simulink model "SPM_Model"  (R2023a)
settings: Solver=ode3  StartTime=0  StopTime=fin  FixedStep=st  MaxStep=0.5  RelTol=1e-3  EnableMultiTasking=on
values from neighbouring files (symbols this model uses):
  Asys_n = alpha1_n * a_setup    [SPM_Script.m]
  Asys_p = alpha1_p * a_setup    [SPM_Script.m]
  Bsys_n = alpha2_n * [zeros(num-1,1); -sr / (sr - 1)]    [SPM_Script.m]
  Bsys_p = alpha2_p * [zeros(num-1,1); -sr / (sr - 1)]    [SPM_Script.m]
  cs_init_n = x_init * cs_max_n    [SPM_Script.m]    (also in TPM_Script.m = (SOC_p20 * (x100_percent_n - x0_percent_n) + x0_percent_n) *)
  cs_init_p = y_init * cs_max_p    [SPM_Script.m]    (also in TPM_Script.m = (SOC_p20 * (y100_percent_p - y0_percent_p) + y0_percent_p) *)
  Csys_n = [zeros(1, num-1), 1]    [SPM_Script.m]
  Csys_p = [zeros(1, num-1), 1]    [SPM_Script.m]
  Dsys_n = -alpha2_n / alpha1_n    [SPM_Script.m]
  Dsys_p = -alpha2_p / alpha1_p    [SPM_Script.m]
  PA = 5    [SPM_Script.m]    (also in TPM_Script.m)
  par = zeros(11, 1)    [TPM_Script.m]
settings Model: Creator=Cra  LastModifiedBy=srose
settings SolverCC: AlgebraicLoopSolver=TrustRegion
settings DataIOCC: SaveFormat=Array  SignalLoggingSaveFormat=ModelDataLogs  SaveOutput=off  SignalLogging=off  ReturnWorkspaceOutputs=off
settings OptimizationCC: ExpressionDepthLimit=2147483647  InitFltsAndDblsToZero=on  LifeSpan=inf
settings DebuggingCC: SaveWithParameterizedLinksMsg=none  UnderspecifiedInitializationDetection=Classic  MergeDetectMultiDrivingBlocksExec=none  SolverPrmCheckMsg=warning  FcnCallInpInsideContextMsg=warning  UnconnectedInputMsg=warning  UnconnectedOutputMsg=warning  UnconnectedLineMsg=warning  StateNameClashWarn=warning  SFUnexpectedBacktrackingDiag=warning  SFNoUnconditionalDefaultTransitionDiag=warning  SFExecutionAtInitializationDiag=none  ArithmeticOperatorsInVariantConditions=warning
settings HardwareCC: ProdBitPerPointer=32  ProdBitPerSizeT=32  ProdBitPerPtrDiffT=32  ProdLargestAtomicFloat=None  ProdIntDivRoundTo=Undefined  ProdEndianess=Unspecified  ProdWordSize=32  ProdHWDeviceType=32-bit Generic
settings ModelReferenceCC: EnableRefExpFcnMdlSchedulingChecks=on  PropagateSignalLabelsOutOfModel=off
settings SFSimCC: SimUseLocalCustomCode=off  CustomCodeUndefinedFunction=UseInterfaceOnly
settings RTWCC: RTWUseLocalCustomCode=off  DLArmComputeVersion=19.05
settings CodeAppCC: StateflowObjectComments=on
settings GRTTargetCC: TargetFcnLib=ansi_tfl_tmw.mat  TargetLangStandard=C89/C90 (ANSI)  CombineOutputUpdateFcns=off  GRTInterface=on
settings ConfigComp: CovMetricSettings=dw  CovSaveCumulativeToWorkspaceVar=on  CovSaveSingleToWorkspaceVar=on  CovExternalEMLEnable=off

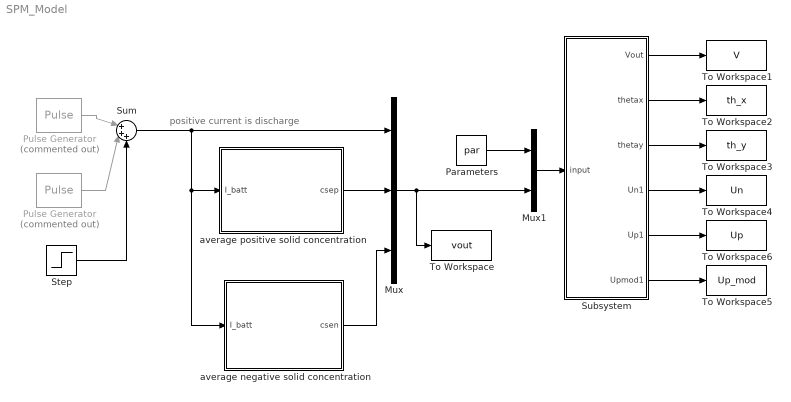
== system SPM_Model ==
  note: positive current is discharge
  Mux : Mux  Inputs=3
  Mux1 : Mux  Inputs=2
  Parameters : Constant  Value=par  VectorParams1D=off
  Pulse Generator : DiscretePulseGenerator  Commented=on  PulseType=Time based  Amplitude=-2*PA  Period=100  PulseWidth=25  PhaseDelay=140
  "Pulse Generator " : DiscretePulseGenerator  Commented=on  PulseType=Time based  Amplitude=PA  Period=100  PulseWidth=25  PhaseDelay=40
  Step : Step  Time=0  After=5  SampleTime=0
  Subsystem : Subsystem
  Sum : Sum  Inputs=|+++
  To Workspace : ToWorkspace  VariableName=vout  SampleTime=-1
  To Workspace1 : ToWorkspace  VariableName=V  SampleTime=-1
  To Workspace2 : ToWorkspace  VariableName=th_x  SampleTime=-1
  To Workspace3 : ToWorkspace  VariableName=th_y  SampleTime=-1
  To Workspace4 : ToWorkspace  VariableName=Un  SampleTime=-1
  To Workspace5 : ToWorkspace  VariableName=Up_mod  SampleTime=-1
  To Workspace6 : ToWorkspace  VariableName=Up  SampleTime=-1
  "average negative solid concentration  " : Subsystem
  average positive solid concentration : Subsystem
  wires:
  average positive solid concentration/1(csep) -> Mux/2
  Mux/1 -> Mux1/2, To Workspace/1
  "average negative solid concentration  "/1(csen) -> Mux/3
  Sum/1 -> average positive solid concentration/1(I_batt), "average negative solid concentration  "/1(I_batt), Mux/1
  "Pulse Generator "/1 -> Sum/1
  Pulse Generator/1 -> Sum/2
  Step/1 -> Sum/3
  Parameters/1 -> Mux1/1
  Mux1/1 -> Subsystem/1(input)
  Subsystem/1(Vout) -> To Workspace1/1
  Subsystem/2(thetax) -> To Workspace2/1
  Subsystem/3(thetay) -> To Workspace3/1
  Subsystem/4(Un1) -> To Workspace4/1
  Subsystem/5(Up1) -> To Workspace6/1
  Subsystem/6(Upmod1) -> To Workspace5/1

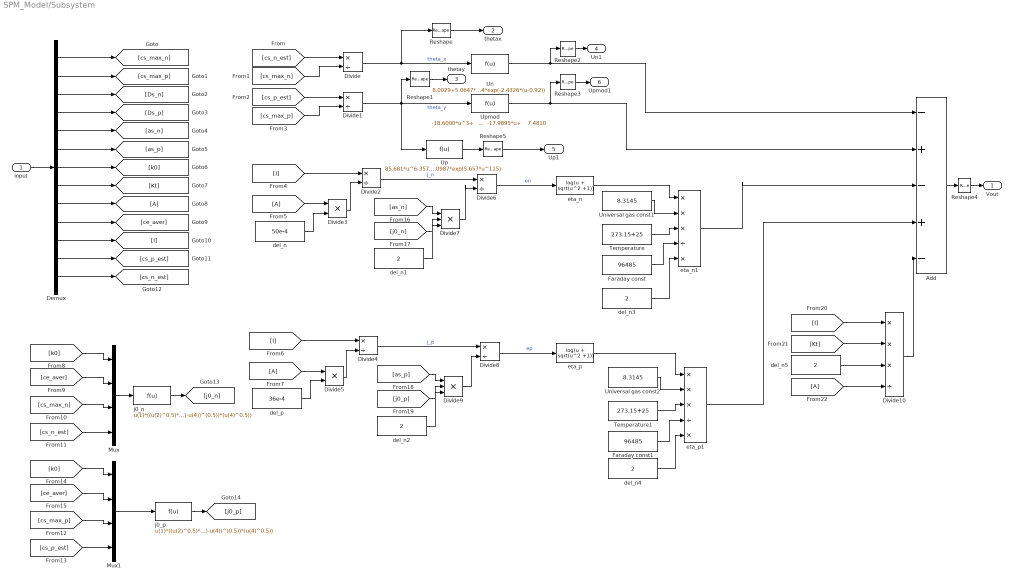
== system SPM_Model/Subsystem ==
  input : Inport
  Add : Sum  Inputs=-+-+-  OutDataTypeStr=double
  Demux : Demux  Outputs=13
  Divide{,1..2,4,6,8} (6 alike) : Product  Inputs=*/
  Divide10 : Product  Inputs=***/
  Divide3 : Product  Inputs=**
  Divide5 : Product  Inputs=**
  Divide7 : Product  Inputs=***
  Divide9 : Product  Inputs=***
  Faraday const : Constant  Value=96485
  Faraday const1 : Constant  Value=96485
  From22 : From
  From5 : From
  From7 : From
  Goto8 : Goto
  Mux : Mux
  Mux1 : Mux
  Reshape{,1..5} (6 alike) : Reshape
  Temperature : Constant  Value=273.15+25
  Temperature1 : Constant  Value=273.15+25
  Un : Fcn  Expr=8.0029+5.0647*u-12.578*u^0.5-8.6322e-4*u^(-1)+2.1765e-5*u^(3/2)-0.46016*exp(15.0*(0.06-u))-0.55364*exp(-2.4326*(u-0.92))
  Universal gas const1 : Constant  Value=8.3145  VectorParams1D=off
  Universal gas const2 : Constant  Value=8.3145
  Up : Fcn  Expr=85.681*u^6-357.70*u^5+613.89*u^4-555.65*u^3+281.06*u^2-76.648*u+13.1983 -0.30987*exp(5.657*u^115)
  Upmod : Fcn  Expr="-18.6000*u^3+   31.1854*u^2  -17.9895*u+    7.4810"
  del_n : Constant  Value=50e-4
  del_n{1..5} (5 alike) : Constant  Value=2
  del_p : Constant  Value=36e-4
  eta_n : Fcn  Expr=log(u + sqrt(u^2 +1))
  eta_n1 : Product  Inputs=***/*
  eta_p : Fcn  Expr=log(u + sqrt(u^2 +1))
  eta_p1 : Product  Inputs=***/*
  j0_n : Fcn  Expr=u(1)*((u(2)^0.5)*((u(3)-u(4))^(0.5))*(u(4)^0.5))
  j0_p : Fcn  Expr=u(1)*((u(2)^0.5)*((u(3)-u(4))^(0.5))*(u(4)^0.5))
  Vout : Outport
  thetax : Outport  Port=2
  thetay : Outport  Port=3
  Un1 : Outport  Port=4
  Up1 : Outport  Port=5
  Upmod1 : Outport  Port=6
  wires:
  input/1 -> Demux/1
  Demux/1 -> [cs_max_n]
  Demux/2 -> [cs_max_p]
  Demux/3 -> [Ds_n]
  Demux/4 -> [Ds_p]
  Demux/5 -> [as_n]
  Demux/6 -> [as_p]
  Demux/7 -> [k0]
  Demux/8 -> [Kt]
  Demux/9 -> Goto8/1
  Demux/10 -> [ce_aver]
  Demux/11 -> [I]
  Demux/12 -> [cs_p_est]
  Demux/13 -> [cs_n_est]
  [cs_n_est] -> Divide/1
  [cs_max_n] -> Divide/2
  Divide/1 -> Un/1, Reshape/1  "theta_x"
  [cs_p_est] -> Divide1/1
  [cs_max_p] -> Divide1/2
  Divide1/1 -> Upmod/1, Up/1, Reshape1/1  "theta_y"
  [I] -> Divide2/1
  From5/1 -> Divide3/1
  del_n/1 -> Divide3/2
  Divide3/1 -> Divide2/2
  Divide2/1 -> Divide6/1  "j_n"
  [I] -> Divide4/1
  From7/1 -> Divide5/1
  del_p/1 -> Divide5/2
  Divide5/1 -> Divide4/2
  Divide4/1 -> Divide8/1  "j_p"
  [k0] -> Mux/1
  [ce_aver] -> Mux/2
  [cs_max_n] -> Mux/3
  [cs_n_est] -> Mux/4
  Mux/1 -> j0_n/1
  [k0] -> Mux1/1
  [ce_aver] -> Mux1/2
  [cs_max_p] -> Mux1/3
  [cs_p_est] -> Mux1/4
  Mux1/1 -> j0_p/1
  [as_n] -> Divide7/1
  [j0_n] -> Divide7/2
  Divide7/1 -> Divide6/2
  j0_n/1 -> [j0_n]
  j0_p/1 -> [j0_p]
  del_n1/1 -> Divide7/3
  [as_p] -> Divide9/1
  [j0_p] -> Divide9/2
  Divide9/1 -> Divide8/2
  del_n2/1 -> Divide9/3
  Divide6/1 -> eta_n/1  "en"
  Divide8/1 -> eta_p/1  "ep"
  Universal gas const1/1 -> eta_n1/2
  Temperature/1 -> eta_n1/3
  Faraday const/1 -> eta_n1/4
  Universal gas const2/1 -> eta_p1/2
  Temperature1/1 -> eta_p1/3
  Faraday const1/1 -> eta_p1/4
  del_n4/1 -> eta_p1/5
  eta_p/1 -> eta_p1/1
  del_n3/1 -> eta_n1/5
  eta_n/1 -> eta_n1/1
  Un/1 -> Add/1, Reshape2/1
  Upmod/1 -> Add/2, Reshape3/1
  eta_n1/1 -> Add/3
  eta_p1/1 -> Add/4
  [I] -> Divide10/1
  [Kt] -> Divide10/2
  del_n5/1 -> Divide10/3
  From22/1 -> Divide10/4
  Divide10/1 -> Add/5
  Add/1 -> Reshape4/1
  Up/1 -> Reshape5/1
  Reshape/1 -> thetax/1
  Reshape1/1 -> thetay/1
  Reshape2/1 -> Un1/1
  Reshape3/1 -> Upmod1/1
  Reshape4/1 -> Vout/1
  Reshape5/1 -> Up1/1

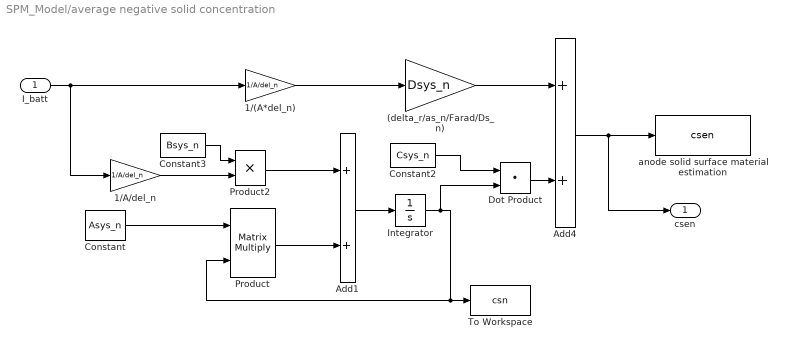
== system SPM_Model/average negative solid concentration   ==
  I_batt : Inport
  (delta_r/as_n/Farad/Ds_n) : Gain  Gain=Dsys_n
  1/(A*del_n) : Gain  Gain=1/A/del_n
  1/A/del_n : Gain  Gain=1/A/del_n
  Add1 : Sum
  Add4 : Sum
  Constant : Constant  Value=Asys_n
  Constant2 : Constant  Value=Csys_n
  Constant3 : Constant  Value=Bsys_n
  Dot Product : DotProduct  OutDataTypeStr=Inherit: Inherit via internal rule
  Integrator : Integrator  InitialCondition=cs_init_n
  Product : Product  Multiplication=Matrix(*)  RndMeth=Zero
  Product2 : Product  RndMeth=Zero
  To Workspace : ToWorkspace  VariableName=csn  SampleTime=-1
  anode solid surface material estimation : ToWorkspace  VariableName=csen  SampleTime=-1
  csen : Outport
  wires:
  Integrator/1 -> Dot Product/2, Product/2, To Workspace/1
  Add1/1 -> Integrator/1
  Constant/1 -> Product/1
  Product/1 -> Add1/2
  Dot Product/1 -> Add4/2
  (delta_r/as_n/Farad/Ds_n)/1 -> Add4/1
  Add4/1 -> anode solid surface material estimation/1, csen/1
  I_batt/1 -> 1/A/del_n/1, 1/(A*del_n)/1
  Constant3/1 -> Product2/1
  Product2/1 -> Add1/1
  1/A/del_n/1 -> Product2/2
  1/(A*del_n)/1 -> (delta_r/as_n/Farad/Ds_n)/1
  Constant2/1 -> Dot Product/1

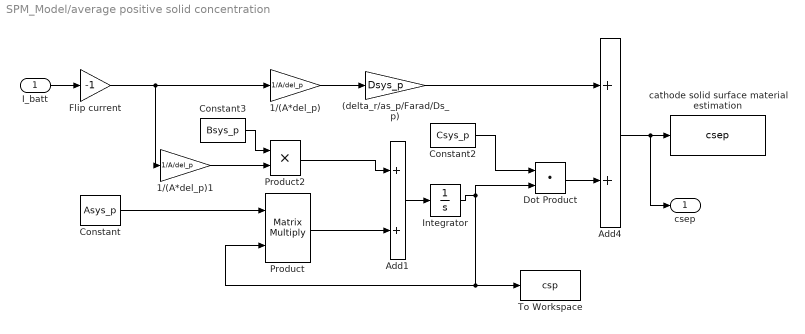
== system SPM_Model/average positive solid concentration ==
  I_batt : Inport
  (delta_r/as_p/Farad/Ds_p) : Gain  Gain=Dsys_p
  1/(A*del_p) : Gain  Gain=1/A/del_p
  1/(A*del_p)1 : Gain  Gain=1/A/del_p
  Add1 : Sum
  Add4 : Sum
  Constant : Constant  Value=Asys_p
  Constant2 : Constant  Value=Csys_p
  Constant3 : Constant  Value=Bsys_p
  Dot Product : DotProduct  OutDataTypeStr=Inherit: Inherit via internal rule
  Flip current : Gain  Gain=-1
  Integrator : Integrator  InitialCondition=cs_init_p  LimitOutput=on
  Product : Product  Multiplication=Matrix(*)  RndMeth=Zero
  Product2 : Product  RndMeth=Zero
  To Workspace : ToWorkspace  VariableName=csp  SampleTime=-1
  cathode solid surface material estimation : ToWorkspace  VariableName=csep  SampleTime=-1
  csep : Outport
  wires:
  Constant2/1 -> Dot Product/1
  1/(A*del_p)/1 -> (delta_r/as_p/Farad/Ds_p)/1
  1/(A*del_p)1/1 -> Product2/2
  Product2/1 -> Add1/1
  Constant3/1 -> Product2/1
  Add4/1 -> cathode solid surface material estimation/1, csep/1
  (delta_r/as_p/Farad/Ds_p)/1 -> Add4/1
  Dot Product/1 -> Add4/2
  Product/1 -> Add1/2
  Constant/1 -> Product/1
  Add1/1 -> Integrator/1
  Integrator/1 -> Dot Product/2, Product/2, To Workspace/1
  Flip current/1 -> 1/(A*del_p)/1, 1/(A*del_p)1/1
  I_batt/1 -> Flip current/1
